simulink model "w31_v6"  (Simulink 7.9)
settings: Solver=FixedStepDiscrete  StartTime=0.0  StopTime=inf  FixedStep=0.01  RelTol=1e-3
undefined symbols (not defined in the file): DiscIntNeverNeededParam, magnitude
libraries: canmsglib x24, cansrvlib x22, simulink x12, iohwablib x5, legionoslib x3, ccpsrvlib x2, memsrvlib x1, tgttoollib x1, udssrvlib x1, wdgmlib x1
(part 3 of 5)

== system w31_v6/CAN_Receive_10ms/Remote_Control_CAN/remote_shake1 ==
  note: 内侧车轮转角30度，此处以内侧车轮为准，所以输出车轮转角为-30度到+30度
      | 车速范围为0-80km/h，纵向控制遥感往前推是加速
      | 制动压力范围0-8mpa，纵向控制遥感往后推是制动
  msg : Inport
  Function : TriggerPort  TriggerType=function-call  PortDimensions=1
  Accelerate : Subsystem  TreatAsAtomicUnit=on
  Constant : Constant  OutDataTypeStr=uint8  SampleTime=-1
  Decelerate : Subsystem  TreatAsAtomicUnit=on
  Gain : Gain  Gain=30/450
  If : If
  Memory : Memory  InheritSampleTime=on
  Merge : Merge
  Merge1 : Merge
  Remote_control_Io : canmsglib/CAN Unpack  CANdbFile=E:\matlab_ws\2012_Matlab_Vcu\w_serial\w3\w32\dbc\w32_CAN1_500kbs_0309_v5.dbc  MsgList=Remote_Control_Shake_2  MsgName=Remote_Control_Shake_2  MsgIDType=Standard (11-bit identifier)  MsgIdentifier=267  MsgLength=8  SignalInfo=Remote_X1_Reserved$48$16$1$1$1$0$1$0$-450$450$#Remote_X2_Lateral_Control$0$16$1$1$1$0$1$0$-450$450$#Remote_Y1_Longitudinal_Control$32$16$1$1$1$0$1$0$-450$450$#Remote_Y2_Reserved$16$16$1$1$1$0$-1$0$-450$450$#  NSignals=4  IDPort=off  TimestampPort=off  ErrorPort=off  RemotePort=off  LengthPort=off  StatusPort=off  StartBits=str2num('[int32(48);int32(0);int32(32);int32(16)]')  SignalSizes=str2num('[int32(16);int32(16);int32(16);int32(16)]')  ByteOrders=str2num('[int32(1);int32(1);int32(1);int32(1)]')  DataTypes=str2num('[int32(1);int32(1);int32(1);int32(1)]')  MultiplexTypes=str2num('[int32(1);int32(1);int32(1);int32(1)]')  MultiplexValues=str2num('[double(0);double(0);double(0);double(0)]')  Factors=str2num('[double(1);double(1);double(1);double(-1)]')  Offsets=str2num('[double(0);double(0);double(0);double(0)]')  Minimums=str2num('[double(-450);double(-450);double(-450);double(-450)]')  Maximums=str2num('[double(450);double(450);double(450);double(450)]')
      settings: DataFormat=CANdb specified signals
  Sum : Sum  Inputs=|++  OutDataTypeStr=uint8
  Terminator1 : Terminator
  Terminator3 : Terminator
  Remote_Power_Required : Outport
  Remote_Brake_Pressure_Required : Outport  Port=2
  Remote_Steering_Angle_Required : Outport  Port=3
  Remote_stutas : Outport  Port=4
  wires:
  Memory/1 -> Sum/2
  Sum/1 -> Memory/1, Remote_stutas/1
  Constant/1 -> Sum/1
  msg/1 -> Remote_control_Io/1
  Remote_control_Io/1 -> Terminator3/1
  Remote_control_Io/2 -> Gain/1
  Gain/1 -> Remote_Steering_Angle_Required/1
  Remote_control_Io/3 -> Accelerate/1(Speed_Required), Decelerate/1(BrakePressureRequired), If/1
  If/1 -> Accelerate/Action
  If/2 -> Decelerate/Action
  Accelerate/1(RemoteSpeedRequired) -> Merge/1
  Decelerate/1(RemoteSpeedRequired) -> Merge/2
  Accelerate/2(RemoteBrakePressureRequired) -> Merge1/1
  Decelerate/2(RemoteBrakePressureRequired) -> Merge1/2
  Merge/1 -> Remote_Power_Required/1
  Merge1/1 -> Remote_Brake_Pressure_Required/1
  Remote_control_Io/4 -> Terminator1/1

== system w31_v6/CAN_Receive_10ms/Remote_Control_CAN/shake_situation1 ==
  note: 输出1表示信号丢失
      | 输出0表示一切正常
  RxMsgCnt : Inport
  NoRxMsgCntMax : Inport  Port=2
  Chart : Stateflow chart  TreatAsAtomicUnit=on
  Relational Operator1 : RelationalOperator  Operator=~=  OutDataTypeStr=boolean
  Terminator : Terminator
  Unit Delay1 : UnitDelay  SampleTime=-1
  NoRxMsgComfirm : Outport
  wires:
  NoRxMsgCntMax/1 -> Chart/2(NoRxMsgCntMax)
  Unit Delay1/1 -> Relational Operator1/1
  RxMsgCnt/1 -> Relational Operator1/2, Unit Delay1/1
  Relational Operator1/1 -> Chart/1(RxMsg)
  Chart/1(NoRxMsgComfirm) -> NoRxMsgComfirm/1
  Chart/2(NoRxMsgCnt) -> Terminator/1

== system w31_v6/CAN_Receive_10ms/Status_Cal/Subsystem ==
  note: 等于0则说明存在严重故障
  Remote : Inport
  Chassis : Inport  Port=2
  iECU : Inport  Port=3
  Hardware : Inport  Port=4
  Bus Creator : BusCreator  Inputs=1
  Bus Creator1 : BusCreator
  Bus Creator2 : BusCreator  Inputs=7
  Bus Creator3 : BusCreator  Inputs=1
  Bus Creator4 : BusCreator  Inputs=2
  Bus Selector : BusSelector  OutputSignals=Remote_Analog.Remote_Analog_Status,Remote_IO.Remote_IO_Status
  Bus Selector1 : BusSelector  OutputSignals=EPSF_Receive.EPSF_Status_NoRxMsg,EPSR_Receive.EPSR_Status_NoRxMsg,DBSF_Receive.DBSF_Status_NoRxMsg,FL_Motor_Receive.FL_Motor_Status_NoRxMsg,FR_Motor_Receive.FR_Motor_Status_NoRxMsg,RL_Motor_Receive.RL_Motor_Status_NoRxMsg,RR_Motor_Receive.RR_Motor_Status_NoRxMsg
  Bus Selector2 : BusSelector  OutputSignals=iECU_Status
  Bus Selector3 : BusSelector  OutputSignals=Key_Ig_Cmd,Eme_Stop_Cmd
  Compare To Zero : simulink/Logic and Bit Operations/Compare To Zero  relop===  OutDataTypeStr=uint8
  Logical Operator : Logic  Operator=OR  AllPortsSameDT=off  OutDataTypeStr=boolean
  Logical Operator1 : Logic  Operator=OR  Inputs=11  AllPortsSameDT=off  OutDataTypeStr=boolean
  Vehicle_State : Outport
  Vehicle_Ready : Outport  Port=2
  wires:
  Remote/1 -> Bus Selector/1
  Bus Selector/1 -> Logical Operator/1  "<Remote_Analog_Status>"
  Bus Selector/2 -> Logical Operator/2  "<Remote_IO_Status>"
  Chassis/1 -> Bus Selector1/1
  Logical Operator/1 -> Bus Creator/1, Logical Operator1/1  "Remote_Status"
  Bus Selector1/1 -> Bus Creator2/1, Logical Operator1/2  "<EPSF_Status_NoRxMsg>"
  Bus Selector1/2 -> Bus Creator2/2, Logical Operator1/3  "<EPSR_Status_NoRxMsg>"
  Bus Selector1/3 -> Bus Creator2/3, Logical Operator1/4  "<DBSF_Status_NoRxMsg>"
  Bus Selector1/4 -> Bus Creator2/5, Logical Operator1/6  "<FL_Motor_Status_NoRxMsg>"
  Bus Selector1/5 -> Bus Creator2/6, Logical Operator1/7  "<FR_Motor_Status_NoRxMsg>"
  Bus Selector1/6 -> Bus Creator2/7, Logical Operator1/8  "<RL_Motor_Status_NoRxMsg>"
  Bus Selector1/7 -> Logical Operator1/9, Bus Creator2/4  "<RR_Motor_Status_NoRxMsg>"
  iECU/1 -> Bus Selector2/1
  Bus Selector2/1 -> Bus Creator3/1, Logical Operator1/10  "<iECU_Status>"
  Hardware/1 -> Bus Selector3/1
  Bus Selector3/1 -> Bus Creator4/1, Compare To Zero/1  "<Key_Ig_Cmd>"
  Bus Selector3/2 -> Bus Creator4/2, Logical Operator1/5  "<Eme_Stop_Cmd>"
  Bus Creator/1 -> Bus Creator1/1  "Remote_Status"
  Bus Creator2/1 -> Bus Creator1/2  "Chassis_Status"
  Bus Creator3/1 -> Bus Creator1/3  "iECU_Status"
  Bus Creator4/1 -> Bus Creator1/4  "Hardware_Status"
  Bus Creator1/1 -> Vehicle_State/1
  Compare To Zero/1 -> Logical Operator1/11
  Logical Operator1/1 -> Vehicle_Ready/1

== system w31_v6/CAN_Receive_10ms/Status_Cal/Subsystem1 ==
  Vehicle_Ready : Inport
  Chassis : Inport  Port=2
  Hardware : Inport  Port=3
  Abs{,1..3} (4 alike) : Abs
  Add1 : Sum  Inputs=++++
  Bus Creator : BusCreator  Inputs=6
  Bus Selector1 : BusSelector  OutputSignals=EPSF_Receive.F_Tire_Angle_Feedback,EPSR_Receive.R_Tire_Angle_Feedback,DBSF_Receive.DBSF_HP_Pressure_Feedback,FL_Motor_Receive.FL_RPM_Feedback,FR_Motor_Receive.FR_RPM_Feedback,RL_Motor_Receive.RL_RPM_Feedback,RR_Motor_Receive.RR_RPM_Feedback
  Bus Selector3 : BusSelector  OutputSignals=Key_Ig_Cmd
  Gain1 : Gain  Gain=1/4
  To_rpm : Gain  Gain=(3.14*0.69*60)/1000
  Vehicle_Status : Outport
  wires:
  Hardware/1 -> Bus Selector3/1
  Chassis/1 -> Bus Selector1/1
  Bus Selector1/1 -> Bus Creator/2  "<F_Tire_Angle_Feedback>"
  Bus Selector1/2 -> Bus Creator/3  "<R_Tire_Angle_Feedback>"
  Bus Selector1/4 -> Abs/1  "<FL_RPM_Feedback>"
  Bus Selector1/5 -> Abs1/1  "<FR_RPM_Feedback>"
  Bus Selector1/6 -> Abs2/1  "<RL_RPM_Feedback>"
  Bus Selector1/7 -> Abs3/1  "<RR_RPM_Feedback>"
  Abs/1 -> Add1/1
  Abs1/1 -> Add1/2
  Abs2/1 -> Add1/3
  Abs3/1 -> Add1/4
  Add1/1 -> Gain1/1
  Gain1/1 -> To_rpm/1
  To_rpm/1 -> Bus Creator/5  "Vehicle_Speed"
  Vehicle_Ready/1 -> Bus Creator/1  "Vehicle_Ready"
  Bus Selector3/1 -> Bus Creator/6  "<Key_Ig_Cmd>"
  Bus Creator/1 -> Vehicle_Status/1
  Bus Selector1/3 -> Bus Creator/4  "<DBSF_HP_Pressure_Feedback>"

== system w31_v6/CAN_Receive_10ms/iECU_CAN/iECU ==
  note: 内侧车轮转角30度，此处以内侧车轮为准，所以输出车轮转角为-30度到+30度
      | 车速范围为0-80km/h，纵向控制遥感往前推是加速
      | 制动压力范围0-8mpa，纵向控制遥感往后推是制动
  msg : Inport
  Function : TriggerPort  TriggerType=function-call  PortDimensions=1
  Constant : Constant  OutDataTypeStr=uint8  SampleTime=-1
  Data Type Conversion1 : DataTypeConversion  OutDataTypeStr=uint8
  Data Type Conversion2 : DataTypeConversion  OutDataTypeStr=uint8
  Data Type Conversion3 : DataTypeConversion  OutDataTypeStr=double
  Data Type Conversion4 : DataTypeConversion  OutDataTypeStr=double
  Memory : Memory  InheritSampleTime=on
  Sum : Sum  Inputs=|++  OutDataTypeStr=uint8
  Terminator : Terminator
  Terminator1 : Terminator
  Terminator2 : Terminator
  iECU_Input : canmsglib/CAN Unpack  CANdbFile=D:\W31_workspace\w31_CAN1_500kbs_0618_v5.1.dbc  MsgList=iECU  MsgName=iECU  MsgIDType=Standard (11-bit identifier)  MsgIdentifier=268  MsgLength=8  SignalInfo=iECU_BrakePressure_Cmd$28$8$1$2$1$0$1.000000e-01$0$0$8$#iECU_Control_Request_Flag$0$1$1$2$1$0$1$0$0$1$#iECU_E_Gear_Request$1$2$1$2$1$0$1$0$0$2$#iECU_FTire_Angle_Cmd$8$10$1$2$1$0$1.000000e-01$-30$-30$30$#iECU_RTire_Angle_Cmd$18$10$1$2$1$0$1.000000e-01$-30$-30$30$#iECU_Reseved1$3$2$1$2$1$0$1$0$0$2$#iECU_Reseved2$5$3$1$2$1$0$1$0$0$7$#iECU_Reseved3$46$18$1$2$1$0$1$0$0$500$#iECU_Speed_Cmd$36$10$1$2$1$0$1.000000e-01$0$0$80$#  NSignals=9  IDPort=off  TimestampPort=off  ErrorPort=off  RemotePort=off  LengthPort=off  StatusPort=off  StartBits=str2num('[int32(28);int32(0);int32(1);int32(8);int32(18);int32(3);int32(5);int32(46);int32(36)]')  SignalSizes=str2num('[int32(8);int32(1);int32(2);int32(10);int32(10);int32(2);int32(3);int32(18);int32(10)]')  ByteOrders=str2num('[int32(1);int32(1);int32(1);int32(1);int32(1);int32(1);int32(1);int32(1);int32(1)]')  DataTypes=str2num('[int32(2);int32(2);int32(2);int32(2);int32(2);int32(2);int32(2);int32(2);int32(2)]')  MultiplexTypes=str2num('[int32(1);int32(1);int32(1);int32(1);int32(1);int32(1);int32(1);int32(1);int32(1)]')  MultiplexValues=str2num('[double(0);double(0);double(0);double(0);double(0);double(0);double(0);double(0);double(0)]')  Factors=str2num('[double(1.000000e-01);double(1);double(1);double(1.000000e-01);double(1.000000e-01);double(1);double(1);double(1);double(1.000000e-01)]')  Offsets=str2num('[double(0);double(0);double(0);double(-30);double(-30);double(0);double(0);double(0);double(0)]')  Minimums=str2num('[double(0);double(0);double(0);double(-30);double(-30);double(0);double(0);double(0);double(0)]')  Maximums=str2num('[double(8);double(1);double(2);double(30);double(30);double(2);double(7);double(500);double(80)]')
      settings: DataFormat=CANdb specified signals
  iECU_Brake_Pressure_Required : Outport
  iECU_Control_Flag : Outport  Port=2
  iECU_Gear_Required : Outport  Port=3
  iECU_FTire_Angle_Required : Outport  Port=4
  iECU_RTire_Angle_Required : Outport  Port=5
  iECU_Speed_Required : Outport  Port=6
  iECU_Stutas : Outport  Port=7
  wires:
  Memory/1 -> Sum/2
  Sum/1 -> Memory/1, iECU_Stutas/1
  Constant/1 -> Sum/1
  msg/1 -> iECU_Input/1
  Data Type Conversion1/1 -> iECU_Control_Flag/1
  Data Type Conversion2/1 -> iECU_Gear_Required/1
  Data Type Conversion3/1 -> iECU_FTire_Angle_Required/1
  Data Type Conversion4/1 -> iECU_RTire_Angle_Required/1
  iECU_Input/1 -> iECU_Brake_Pressure_Required/1  "iECU_Brake_Pressure_Required"
  iECU_Input/2 -> Data Type Conversion1/1  "iECU_Control_Flag"
  iECU_Input/3 -> Data Type Conversion2/1  "iECU_Gear_Required"
  iECU_Input/4 -> Data Type Conversion3/1  "iECU_FTire_Angle_Required"
  iECU_Input/5 -> Data Type Conversion4/1  "iECU_RTire_Angle_Required"
  iECU_Input/6 -> Terminator/1
  iECU_Input/9 -> iECU_Speed_Required/1  "iECU_Speed_Required"
  iECU_Input/7 -> Terminator1/1
  iECU_Input/8 -> Terminator2/1

== system w31_v6/CAN_Receive_10ms/iECU_CAN/shake_situation1 ==
  note: 输出1表示信号丢失
      | 输出0表示一切正常
  RxMsgCnt : Inport
  NoRxMsgCntMax : Inport  Port=2
  Chart : Stateflow chart  TreatAsAtomicUnit=on
  Relational Operator1 : RelationalOperator  Operator=~=  OutDataTypeStr=boolean
  Terminator : Terminator
  Unit Delay1 : UnitDelay  SampleTime=-1
  NoRxMsgComfirm : Outport
  wires:
  NoRxMsgCntMax/1 -> Chart/2(NoRxMsgCntMax)
  Unit Delay1/1 -> Relational Operator1/1
  RxMsgCnt/1 -> Relational Operator1/2, Unit Delay1/1
  Relational Operator1/1 -> Chart/1(RxMsg)
  Chart/1(NoRxMsgComfirm) -> NoRxMsgComfirm/1
  Chart/2(NoRxMsgCnt) -> Terminator/1

== system w31_v6/Logic_And_Algorithm/Remote_mode_with_control_0/Brake_calculation ==
  0_4Mpa : Saturate  UpperLimit=4  LowerLimit=0
  Constant : Constant  SampleTime=-1
  Constant1 : Constant  Value=2  SampleTime=-1
  Constant2 : Constant  Value=0  SampleTime=-1
  Constant3 : Constant  Value=0  SampleTime=-1
  Delay : Delay  DelayLength=100
  Gain : Gain  Gain=2
  Multiport Switch : MultiPortSwitch  DataPortOrder=Specify indices  DataPortIndices={0,2,1}  zeroidx=off
  Sum : Sum  Inputs=|++
  Switch : Switch  Criteria=u2 > Threshold
  Break_Req : Outport
  Remote_EPB_Req : Outport  Port=2
  wires:
  [Remote_Brake_Pressure_Required_0] -> Sum/1
  Gain/1 -> Sum/2
  Sum/1 -> 0_4Mpa/1
  0_4Mpa/1 -> Break_Req/1  "Break_Req"
  [No_Remote_CAN_Msg_Or_Emg_Button_0] -> Gain/1
  [EPB_Control_Mode_0] -> Multiport Switch/1
  Constant/1 -> Multiport Switch/2
  Constant1/1 -> Multiport Switch/3
  Constant2/1 -> Multiport Switch/4
  Switch/1 -> Remote_EPB_Req/1
  [Key_Ig_Cmd_0] -> Delay/1
  Constant3/1 -> Switch/3
  Multiport Switch/1 -> Switch/1  "Remote_EPB_Req"
  Delay/1 -> Switch/2

== system w31_v6/Logic_And_Algorithm/Remote_mode_with_control_0/Power_calculation ==
  note: 输入是前进、倒退，输出是四个电机分别的旋转方向
  Constant : Constant  OutDataTypeStr=uint8
  Constant1 : Constant  Value=-1  OutDataTypeStr=int16
  Constant2 : Constant  Value=0  OutDataTypeStr=uint8
  Data Type Conversion : DataTypeConversion  OutDataTypeStr=uint8
  Display{,1..3} (4 alike) : Display
  Multiport Switch : MultiPortSwitch  DataPortOrder=Specify indices  DataPortIndices={0,2,1}  zeroidx=off  OutDataTypeStr=double
  PID_Controller : Subsystem
  Product{,1..3} (4 alike) : Product  RndMeth=Zero
  Speed distribution strategy : Subsystem
  Power_FL : Outport
  Power_FR : Outport  Port=2
  Power_RL : Outport  Port=3
  Power_RR : Outport  Port=4
  wires:
  [Remote_Gear1_0] -> Data Type Conversion/1
  Data Type Conversion/1 -> Multiport Switch/1, Display2/1
  Constant/1 -> Multiport Switch/2
  Constant1/1 -> Multiport Switch/3
  Constant2/1 -> Multiport Switch/4
  Multiport Switch/1 -> Product/1, Product1/1, Product2/1, Product3/1, Display1/1  "Rotation_to_Motor"
  PID_Controller/1(Power_to_FL) -> Product/2, Display/1  "Power_to_FR_Motor"
  PID_Controller/2(Power_to_FR) -> Product1/2  "Power_to_FL_Motor"
  PID_Controller/3(Power_to_RL) -> Product2/2  "Power_to_RR_Motor"
  PID_Controller/4(Power_to_RR) -> Product3/2  "Power_to_RL_Motor"
  Speed distribution strategy/1(Speed_to_FL_PID) -> PID_Controller/1(Desired_Speed_To_FL)
  Speed distribution strategy/2(Speed_to_FR_PID) -> PID_Controller/2(Desired_Speed_To_FR)
  Speed distribution strategy/3(Speed_to_RL_PID) -> PID_Controller/3(Desired_Speed_To_RL)
  Speed distribution strategy/4(Speed_to_RR_PID) -> PID_Controller/4(Desired_Speed_To_RR)
  Product/1 -> Power_FL/1  "Power_FL"
  Product1/1 -> Power_FR/1  "Power_FR"
  Product2/1 -> Power_RL/1  "Power_RL"
  Product3/1 -> Power_RR/1  "Power_RR"

== system w31_v6/Logic_And_Algorithm/Remote_mode_with_control_0/Signal_Input ==
  Chassis_CAN_input : Inport
  Sensor_CAN_input : Inport  Port=2
  Remote_CAN_input : Inport  Port=3
  Hardware_input : Inport  Port=4
  No_Remote_CAN_Msg_Or_Emg_Button : Inport  Port=5
  Chassis_Signal_Goto : Subsystem
  Emg_No_Msg : Subsystem
  Hardware_Signal_Goto1 : Subsystem
  Remote_Signal_Goto : Subsystem
  Terminator1 : Terminator
  wires:
  Chassis_CAN_input/1 -> Chassis_Signal_Goto/1(Chassis_Receive_input)
  Sensor_CAN_input/1 -> Terminator1/1
  Hardware_input/1 -> Hardware_Signal_Goto1/1(Hardware_input)
  Remote_CAN_input/1 -> Remote_Signal_Goto/1(Remote_CAN_input)
  No_Remote_CAN_Msg_Or_Emg_Button/1 -> Emg_No_Msg/1(No_Remote_CAN_Msg_Or_Emg_Button)

== system w31_v6/Logic_And_Algorithm/Remote_mode_with_control_0/Steering_calculation ==
  note: 前轮转角增大1.2倍
  Angle_Cal : Subsystem
  Angle_Control_Mode1 : Constant  Value=32  OutDataTypeStr=uint8
  F_Angle_Control_Mode : Constant  Value=32  OutDataTypeStr=uint8
  F_Angle_Rate : Constant  Value=500
  R_Angle_Rate : Constant  Value=500
  F_Steering_Angle : Outport
  R_Steering_Angle : Outport  Port=2
  F_Steering_Work_Mode : Outport  Port=3
  R_Steering_Work_Mode : Outport  Port=4
  F_Steering_Angle_Rate : Outport  Port=5
  R_Steering_Angle_Rate : Outport  Port=6
  wires:
  F_Angle_Control_Mode/1 -> F_Steering_Work_Mode/1  "F_Steering_Work_Mode"
  Angle_Cal/1(F_Steering_Angle) -> F_Steering_Angle/1  "F_Steering_Angle"
  Angle_Cal/2(R_Steering_Angle) -> R_Steering_Angle/1  "R_Steering_Angle"
  Angle_Control_Mode1/1 -> R_Steering_Work_Mode/1  "R_Steering_Work_Mode"
  F_Angle_Rate/1 -> F_Steering_Angle_Rate/1  "F_Steering_Angle_Rate"
  R_Angle_Rate/1 -> R_Steering_Angle_Rate/1  "R_Steering_Angle_Rate"

== system w31_v6/Logic_And_Algorithm/Remote_mode_with_control_2/Brake_calculation ==
  0_4Mpa : Saturate  UpperLimit=4  LowerLimit=0
  Compare To Constant : simulink/Logic and Bit Operations/Compare To Constant  relop=>=  const=650  OutDataTypeStr=uint8
  Constant : Constant  SampleTime=-1
  Constant1 : Constant  Value=2  SampleTime=-1
  Constant2 : Constant  Value=0  SampleTime=-1
  Constant3 : Constant  Value=0  SampleTime=-1
  Delay : Delay  DelayLength=100
  Gain : Gain  Gain=2
  Logical Operator : Logic  Operator=OR  AllPortsSameDT=off  OutDataTypeStr=boolean
  Multiport Switch : MultiPortSwitch  DataPortOrder=Specify indices  DataPortIndices={0,2,1}  zeroidx=off
  Sum : Sum  Inputs=|++
  Switch : Switch  Criteria=u2 > Threshold
  Break_Req : Outport
  Remote_EPB_Req : Outport  Port=2
  wires:
  Delay/1 -> Switch/2
  Multiport Switch/1 -> Switch/1  "Remote_EPB_Req"
  Constant3/1 -> Switch/3
  [Key_Ig_Cmd_2] -> Delay/1
  Switch/1 -> Remote_EPB_Req/1
  Constant2/1 -> Multiport Switch/4
  Constant1/1 -> Multiport Switch/3
  Constant/1 -> Multiport Switch/2
  [EPB_Control_Mode_2] -> Multiport Switch/1
  [No_Remote_CAN_Msg_Or_Emg_Button_2] -> Gain/1
  0_4Mpa/1 -> Break_Req/1  "Break_Req"
  Sum/1 -> 0_4Mpa/1
  Gain/1 -> Sum/2
  [Remote_Brake_Pressure_Required_2] -> Sum/1
  [Remote_Power_Required_2] -> Compare To Constant/1
  Compare To Constant/1 -> Logical Operator/1

== system w31_v6/Logic_And_Algorithm/Remote_mode_with_control_2/Power_calculation ==
  note: 输入是前进、倒退，输出是四个电机分别的旋转方向
  Constant : Constant  OutDataTypeStr=double
  Constant1 : Constant  Value=-1  OutDataTypeStr=double
  Constant2 : Constant  Value=0  OutDataTypeStr=double
  Data Type Conversion : DataTypeConversion  OutDataTypeStr=double
  Multiport Switch : MultiPortSwitch  DataPortOrder=Specify indices  DataPortIndices={0,2,1}  zeroidx=off  OutDataTypeStr=double
  PID_Controller : Subsystem
  Product{,1..3} (4 alike) : Product  RndMeth=Zero
  Speed distribution strategy : Subsystem
  Power_FL : Outport
  Power_FR : Outport  Port=2
  Power_RL : Outport  Port=3
  Power_RR : Outport  Port=4
  wires:
  Speed distribution strategy/3(Speed_to_RL_PID) -> PID_Controller/3(Desired_Speed_To_RL)
  Speed distribution strategy/4(Speed_to_RR_PID) -> PID_Controller/4(Desired_Speed_To_RR)
  Speed distribution strategy/1(Speed_to_FL_PID) -> PID_Controller/1(Desired_Speed_To_FL)
  Speed distribution strategy/2(Speed_to_FR_PID) -> PID_Controller/2(Desired_Speed_To_FR)
  [Remote_Gear1_2] -> Data Type Conversion/1
  Constant/1 -> Multiport Switch/2
  Constant1/1 -> Multiport Switch/3
  Constant2/1 -> Multiport Switch/4
  Multiport Switch/1 -> Product/1, Product2/1, Product3/1, Product1/1
  Data Type Conversion/1 -> Multiport Switch/1
  PID_Controller/1(Torque_to_FL_Motor) -> Product/2  "Power_to_FL_Motor"
  PID_Controller/2(Torque_to_FR_Motor) -> Product1/2  "Power_to_FR_Motor"
  Product1/1 -> Power_FR/1  "Power_FR"
  PID_Controller/3(Torque_to_RL_Motor) -> Product2/2  "Power_to_RL_Motor"
  Product2/1 -> Power_RL/1  "Power_RL"
  PID_Controller/4(Torque_to_RR_Motor) -> Product3/2  "Power_to_RR_Motor"
  Product3/1 -> Power_RR/1  "Power_RR"
  Product/1 -> Power_FL/1  "Power_FL"

== system w31_v6/Logic_And_Algorithm/Remote_mode_with_control_2/Signal_Input ==
  Remote_CAN_input : Inport
  Hardware_input : Inport  Port=2
  No_Remote_CAN_Msg_Or_Emg_Button : Inport  Port=3
  Emg_No_Msg : Subsystem
  Hardware_Signal_Goto1 : Subsystem
  Remote_Signal_Goto : Subsystem
  wires:
  No_Remote_CAN_Msg_Or_Emg_Button/1 -> Emg_No_Msg/1(No_Remote_CAN_Msg_Or_Emg_Button)
  Remote_CAN_input/1 -> Remote_Signal_Goto/1(Remote_CAN_input)
  Hardware_input/1 -> Hardware_Signal_Goto1/1(Hardware_input)

== system w31_v6/Logic_And_Algorithm/Remote_mode_with_control_2/Steering_calculation ==
  note: 前轮转角增大1.2倍
  Angle_Cal : Subsystem
  Angle_Control_Mode1 : Constant  Value=32  OutDataTypeStr=uint8
  F_Angle_Control_Mode : Constant  Value=32  OutDataTypeStr=uint8
  F_Angle_Rate : Constant  Value=500
  R_Angle_Rate : Constant  Value=500
  F_Steering_Angle : Outport
  R_Steering_Angle : Outport  Port=2
  F_Steering_Work_Mode : Outport  Port=3
  R_Steering_Work_Mode : Outport  Port=4
  F_Steering_Angle_Rate : Outport  Port=5
  R_Steering_Angle_Rate : Outport  Port=6
  wires:
  R_Angle_Rate/1 -> R_Steering_Angle_Rate/1  "R_Steering_Angle_Rate"
  F_Angle_Rate/1 -> F_Steering_Angle_Rate/1  "F_Steering_Angle_Rate"
  Angle_Control_Mode1/1 -> R_Steering_Work_Mode/1  "R_Steering_Work_Mode"
  Angle_Cal/2(R_Steering_Angle) -> R_Steering_Angle/1  "R_Steering_Angle"
  Angle_Cal/1(F_Steering_Angle) -> F_Steering_Angle/1  "F_Steering_Angle"
  F_Angle_Control_Mode/1 -> F_Steering_Work_Mode/1  "F_Steering_Work_Mode"

== system w31_v6/Logic_And_Algorithm/iECU_mode_with_control/Brake_calculation ==
  0_4Mpa : Saturate  UpperLimit=4  LowerLimit=0
  Gain : Gain  Gain=2
  Sum : Sum  Inputs=|+++
  Break_Req : Outport
  wires:
  [iECU_BrakePressureReq] -> Sum/1
  Sum/1 -> 0_4Mpa/1
  0_4Mpa/1 -> Break_Req/1  "Break_Req"
  [No_iECU_CAN_Msg_Or_Emg_Button] -> Gain/1
  Gain/1 -> Sum/3
  [iECU_RemoteBrakePressure] -> Sum/2

== system w31_v6/Logic_And_Algorithm/iECU_mode_with_control/Power_calculation ==
  note: 输入是前进、倒退，输出是四个电机分别的旋转方向
  Bus Creator1 : BusCreator
  Bus Creator2 : BusCreator
  PID_Controller : Subsystem
  PID_Reset_Cal : Subsystem
  Speed distribution strategy : Subsystem
  Subsystem : Subsystem
  Rotation_to_Motor_CANBus : Outport
  Torque_to_Motor_CANBus : Outport  Port=2
  wires:
  Bus Creator1/1 -> Rotation_to_Motor_CANBus/1  "Rotation_to_Motor_CANBus"
  Bus Creator2/1 -> Torque_to_Motor_CANBus/1  "Torque_to_Motor_CANBus"
  Speed distribution strategy/1(Speed_to_FR_PID) -> PID_Controller/1(Desired_Speed_To_FR)
  Speed distribution strategy/2(Speed_to_FL_PID) -> PID_Controller/2(Desired_Speed_To_FL1)
  Speed distribution strategy/3(Speed_to_RR_PID) -> PID_Controller/3(Desired_Speed_To_RR)
  Speed distribution strategy/4(Speed_to_RL_PID) -> PID_Controller/4(Desired_Speed_To_RL)
  Subsystem/1(Rotation_to_FL_Motor) -> Bus Creator1/1
  Subsystem/2(Rotation_to_FR_Motor) -> Bus Creator1/2
  Subsystem/3(Rotation_to_RL_Motor) -> Bus Creator1/3
  Subsystem/4(Rotation_to_RR_Motor) -> Bus Creator1/4
  PID_Controller/1(Torque_to_FR_Motor) -> Bus Creator2/1  "Torque_to_FR_Motor"
  PID_Controller/2(Torque_to_FL_Motor) -> Bus Creator2/2  "Torque_to_FL_Motor"
  PID_Controller/3(Torque_to_RR_Motor) -> Bus Creator2/3  "Torque_to_RR_Motor"
  PID_Controller/4(Torque_to_RL_Motor) -> Bus Creator2/4  "Torque_to_RL_Motor"

== system w31_v6/Logic_And_Algorithm/iECU_mode_with_control/Signal_Input ==
  Chassis_CAN_input : Inport
  Sensor_CAN_input : Inport  Port=2
  Remote_CAN_input : Inport  Port=3
  Hardware_input : Inport  Port=4
  iECU_CAN_input : Inport  Port=5
  No_iECU_CAN_Msg_Or_Emg_Button : Inport  Port=6
  Emg_No_Msg : Subsystem
  Hardware_Signal_Goto : Subsystem
  Remote_Signal_Goto : Subsystem
  Terminator : Terminator
  Terminator1 : Terminator
  iECU_Signal_Goto : Subsystem
  wires:
  Chassis_CAN_input/1 -> Hardware_Signal_Goto/1(Chassis_Receive_input)
  Sensor_CAN_input/1 -> Terminator1/1
  Hardware_input/1 -> Terminator/1
  Remote_CAN_input/1 -> Remote_Signal_Goto/1(Remote_CAN_input)
  iECU_CAN_input/1 -> iECU_Signal_Goto/1(iECU_CAN_input)
  No_iECU_CAN_Msg_Or_Emg_Button/1 -> Emg_No_Msg/1(No_iECU_CAN_Msg_Or_Emg_Button)

== system w31_v6/Logic_And_Algorithm/iECU_mode_with_control/Steering_calculation ==
  Angle_Control_Mode1 : Constant  Value=32  OutDataTypeStr=uint8
  F_Angle_Control_Mode : Constant  Value=32  OutDataTypeStr=uint8
  F_Angle_Rate : Constant  Value=500
  R_Angle_Rate : Constant  Value=500
  F_Steering_Angle : Outport
  R_Steering_Angle : Outport  Port=2
  F_Steering_Work_Mode : Outport  Port=3
  R_Steering_Work_Mode : Outport  Port=4
  F_Steering_Angle_Rate : Outport  Port=5
  R_Steering_Angle_Rate : Outport  Port=6
  wires:
  F_Angle_Control_Mode/1 -> F_Steering_Work_Mode/1  "F_Steering_Work_Mode"
  Angle_Control_Mode1/1 -> R_Steering_Work_Mode/1  "R_Steering_Work_Mode"
  F_Angle_Rate/1 -> F_Steering_Angle_Rate/1  "F_Steering_Angle_Rate"
  R_Angle_Rate/1 -> R_Steering_Angle_Rate/1  "R_Steering_Angle_Rate"
  [iECU_FTire_Angle_Rrquired] -> F_Steering_Angle/1
  [iECU_RTire_Angle_Rrquired] -> R_Steering_Angle/1

== system w31_v6/10ms_Signal_Output/SteerCAN_Out1/F/Subsystem ==
  deserved_angle : Inport
  Add1 : Sum
  Data Type Conversion : DataTypeConversion  OutDataTypeStr=uint8
  Data Type Conversion1 : DataTypeConversion  OutDataTypeStr=uint8
  Divide2 : Product  Inputs=*/
  Math Function2 : Math  Operator=mod  OutputSignalType=real  SaturateOnIntegerOverflow=on
  eps_angle_base : Constant  Value=256  OutDataTypeStr=double  SampleTime=-1
  eps_angle_init : Constant  Value=1024  OutDataTypeStr=Inherit: Inherit via back propagation  SampleTime=-1
  cmd_angle_high : Outport  OutDataTypeStr=uint8
  cmd_angle_low : Outport  Port=2  OutDataTypeStr=uint8
  wires:
  Add1/1 -> Math Function2/1, Divide2/1
  eps_angle_init/1 -> Add1/2
  eps_angle_base/1 -> Math Function2/2, Divide2/2
  Math Function2/1 -> Data Type Conversion1/1
  Divide2/1 -> Data Type Conversion/1
  Data Type Conversion/1 -> cmd_angle_high/1
  Data Type Conversion1/1 -> cmd_angle_low/1
  deserved_angle/1 -> Add1/1

== system w31_v6/10ms_Signal_Output/SteerCAN_Out1/R/Subsystem ==
  deserved_angle : Inport
  Add1 : Sum
  Data Type Conversion : DataTypeConversion  OutDataTypeStr=uint8
  Data Type Conversion1 : DataTypeConversion  OutDataTypeStr=uint8
  Divide2 : Product  Inputs=*/
  Math Function2 : Math  Operator=mod  OutputSignalType=real  SaturateOnIntegerOverflow=on
  eps_angle_base : Constant  Value=256  OutDataTypeStr=double  SampleTime=-1
  eps_angle_init : Constant  Value=1024  OutDataTypeStr=Inherit: Inherit via back propagation  SampleTime=-1
  cmd_angle_high : Outport  OutDataTypeStr=uint8
  cmd_angle_low : Outport  Port=2  OutDataTypeStr=uint8
  wires:
  Add1/1 -> Math Function2/1, Divide2/1
  eps_angle_init/1 -> Add1/2
  eps_angle_base/1 -> Math Function2/2, Divide2/2
  Math Function2/1 -> Data Type Conversion1/1
  Divide2/1 -> Data Type Conversion/1
  Data Type Conversion/1 -> cmd_angle_high/1
  Data Type Conversion1/1 -> cmd_angle_low/1
  deserved_angle/1 -> Add1/1

== system w31_v6/CAN_Receive_10ms/Hardware_Input/DI signal jittered/DI HS signal jitter1 ==
  DISig : Inport
  Compare To Zero : simulink/Logic and Bit Operations/Compare To Zero  relop=>  OutDataTypeStr=uint8
  Logical Operator : Logic  Inputs=3  AllPortsSameDT=off  OutDataTypeStr=boolean
  Logical Operator1 : Logic  Operator=OR  Inputs=3  AllPortsSameDT=off  OutDataTypeStr=boolean
  Memory{,1,5..6} (4 alike) : Memory  X0=1  InheritSampleTime=on
  Switch : Switch  Criteria=u2 ~= 0
  DISigJittered : Outport
  wires:
  Memory6/1 -> Logical Operator1/3
  Memory1/1 -> Logical Operator/3
  Switch/1 -> DISigJittered/1
  DISig/1 -> Compare To Zero/1
  Memory/1 -> Logical Operator/2, Memory1/1
  Memory5/1 -> Logical Operator1/2, Memory6/1
  Logical Operator/1 -> Switch/1
  Logical Operator1/1 -> Switch/3
  Compare To Zero/1 -> Logical Operator1/1, Memory5/1, Memory/1, Logical Operator/1, Switch/2

== system w31_v6/CAN_Receive_10ms/Hardware_Input/DI signal jittered/DI HS signal jitter2 ==
  DISig : Inport
  Compare To Zero : simulink/Logic and Bit Operations/Compare To Zero  relop=>  OutDataTypeStr=uint8
  Logical Operator : Logic  Inputs=3  AllPortsSameDT=off  OutDataTypeStr=boolean
  Logical Operator1 : Logic  Operator=OR  Inputs=3  AllPortsSameDT=off  OutDataTypeStr=boolean
  Memory{,1,5..6} (4 alike) : Memory  X0=1  InheritSampleTime=on
  Switch : Switch  Criteria=u2 ~= 0
  DISigJittered : Outport
  wires:
  Memory6/1 -> Logical Operator1/3
  Memory1/1 -> Logical Operator/3
  Switch/1 -> DISigJittered/1
  DISig/1 -> Compare To Zero/1
  Memory/1 -> Logical Operator/2, Memory1/1
  Memory5/1 -> Logical Operator1/2, Memory6/1
  Logical Operator/1 -> Switch/1
  Logical Operator1/1 -> Switch/3
  Compare To Zero/1 -> Logical Operator1/1, Memory5/1, Memory/1, Logical Operator/1, Switch/2

== system w31_v6/CAN_Receive_10ms/Hardware_Input/DI signal jittered/DI HS signal jitter3 ==
  DISig : Inport
  Compare To Zero : simulink/Logic and Bit Operations/Compare To Zero  relop=>  OutDataTypeStr=uint8
  Logical Operator : Logic  Inputs=3  AllPortsSameDT=off  OutDataTypeStr=boolean
  Logical Operator1 : Logic  Operator=OR  Inputs=3  AllPortsSameDT=off  OutDataTypeStr=boolean
  Memory{,1,5..6} (4 alike) : Memory  X0=1  InheritSampleTime=on
  Switch : Switch  Criteria=u2 ~= 0
  DISigJittered : Outport
  wires:
  Compare To Zero/1 -> Switch/2, Logical Operator/1, Memory/1, Memory5/1, Logical Operator1/1
  Logical Operator1/1 -> Switch/3
  Logical Operator/1 -> Switch/1
  Memory5/1 -> Memory6/1, Logical Operator1/2
  Memory/1 -> Memory1/1, Logical Operator/2
  DISig/1 -> Compare To Zero/1
  Switch/1 -> DISigJittered/1
  Memory1/1 -> Logical Operator/3
  Memory6/1 -> Logical Operator1/3

== system w31_v6/CAN_Receive_10ms/Hardware_Input/DI signal jittered/DI HS signal jitter8 ==
  DISig : Inport
  Compare To Zero : simulink/Logic and Bit Operations/Compare To Zero  relop=>  OutDataTypeStr=uint8
  Logical Operator : Logic  Inputs=3  AllPortsSameDT=off  OutDataTypeStr=boolean
  Logical Operator1 : Logic  Operator=OR  Inputs=3  AllPortsSameDT=off  OutDataTypeStr=boolean
  Memory{,1,5..6} (4 alike) : Memory  X0=1  InheritSampleTime=on
  Switch : Switch  Criteria=u2 ~= 0
  DISigJittered : Outport
  wires:
  Compare To Zero/1 -> Switch/2, Logical Operator/1, Memory/1, Memory5/1, Logical Operator1/1
  Logical Operator1/1 -> Switch/3
  Logical Operator/1 -> Switch/1
  Memory5/1 -> Memory6/1, Logical Operator1/2
  Memory/1 -> Memory1/1, Logical Operator/2
  DISig/1 -> Compare To Zero/1
  Switch/1 -> DISigJittered/1
  Memory1/1 -> Logical Operator/3
  Memory6/1 -> Logical Operator1/3

== system w31_v6/CAN_Receive_10ms/Remote_Control_CAN/remote_shake1/Accelerate ==
  note: 0-80kph
  Speed_Required : Inport
  Action Port : ActionPort  ActionType=then
  BrakePressureRequired : Constant  Value=0
  Gain : Gain  Gain=30/450
  To_rpm : Gain  Gain=1000/(3.14*0.53*60)
  RemoteSpeedRequired : Outport
  RemoteBrakePressureRequired : Outport  Port=2
  wires:
  BrakePressureRequired/1 -> RemoteBrakePressureRequired/1
  Speed_Required/1 -> Gain/1
  Gain/1 -> To_rpm/1
  To_rpm/1 -> RemoteSpeedRequired/1

== system w31_v6/CAN_Receive_10ms/Remote_Control_CAN/remote_shake1/Decelerate ==
  note: 0-4Mpa
  BrakePressureRequired : Inport
  Action Port : ActionPort  ActionType=else
  Gain : Gain  Gain=-4/450
  SpeedRequired : Constant  Value=0
  RemoteSpeedRequired : Outport
  RemoteBrakePressureRequired : Outport  Port=2
  wires:
  SpeedRequired/1 -> RemoteSpeedRequired/1
  BrakePressureRequired/1 -> Gain/1
  Gain/1 -> RemoteBrakePressureRequired/1

== system w31_v6/Logic_And_Algorithm/Remote_mode_with_control_0/Power_calculation/PID_Controller ==
  note: p调整为1.5
      | i调整为1
  Desired_Speed_To_FL : Inport
  Desired_Speed_To_FR : Inport  Port=2
  Desired_Speed_To_RL : Inport  Port=3
  Desired_Speed_To_RR : Inport  Port=4
  Power_to_FL : Outport
  Power_to_FR : Outport  Port=2
  Power_to_RL : Outport  Port=3
  Power_to_RR : Outport  Port=4
  wires:
  Desired_Speed_To_FL/1 -> Power_to_FL/1
  Desired_Speed_To_FR/1 -> Power_to_FR/1
  Desired_Speed_To_RL/1 -> Power_to_RL/1
  Desired_Speed_To_RR/1 -> Power_to_RR/1

== system w31_v6/Logic_And_Algorithm/Remote_mode_with_control_0/Power_calculation/Speed distribution strategy ==
  Data Type Conversion1 : DataTypeConversion
  Gain : Gain
  MATLAB Function : MATLAB Function  TreatAsAtomicUnit=on
  Switch{,1..3} (4 alike) : Switch  Criteria=u2 ~= 0
  Terminator : Terminator
  Terminator1 : Terminator
  motion distribution1 : Subsystem
  speed gear slection : MATLAB Function  TreatAsAtomicUnit=on
  Speed_to_FL_PID : Outport
  Speed_to_FR_PID : Outport  Port=2
  Speed_to_RL_PID : Outport  Port=3
  Speed_to_RR_PID : Outport  Port=4
  wires:
  [Remote_Gear2_0] -> Data Type Conversion1/1
  [Remote_Power_Required_0] -> speed gear slection/2(u2)
  Data Type Conversion1/1 -> speed gear slection/1(u1)
  motion distribution1/1(motion_f_dem) -> Terminator/1
  motion distribution1/2(motion_r_dem) -> Terminator1/1
  speed gear slection/1(y) -> motion distribution1/1(motion_dem), Gain/1
  [F_Steering_Angle] -> motion distribution1/2(steering angle_f_dem), MATLAB Function/1(delta_f)
  [R_Steering_Angle] -> motion distribution1/3(steering angle_r_dem), MATLAB Function/2(delta_r)
  [steering_mode_0] -> motion distribution1/4(drive mode), MATLAB Function/3(mode)
  motion distribution1/3(motion_fl_dem) -> Switch/3
  motion distribution1/4(motion_fr_dem) -> Switch1/3
  motion distribution1/5(motion_rl_dem) -> Switch2/3
  motion distribution1/6(motion_rr_dem) -> Switch3/3
  MATLAB Function/1(nan_code) -> Switch/2, Switch1/2, Switch2/2, Switch3/2
  Gain/1 -> Switch/1, Switch1/1, Switch2/1, Switch3/1
  Switch/1 -> Speed_to_FL_PID/1
  Switch1/1 -> Speed_to_FR_PID/1
  Switch2/1 -> Speed_to_RL_PID/1
  Switch3/1 -> Speed_to_RR_PID/1

== system w31_v6/Logic_And_Algorithm/Remote_mode_with_control_0/Signal_Input/Chassis_Signal_Goto ==
  Chassis_Receive_input : Inport
  Bus Selector3 : BusSelector  OutputSignals=FL_Motor_Receive.FL_RPM_Feedback,FR_Motor_Receive.FR_RPM_Feedback,RL_Motor_Receive.RL_RPM_Feedback,RR_Motor_Receive.RR_RPM_Feedback,DBSF_Receive.DBSF_Status_NoRxMsg,EPSF_Receive.F_Tire_Angle_Feedback,EPSR_Receive.R_Tire_Angle_Feedback
  tag scope: FL_RPM_Feedback=global, FR_RPM_Feedback=global, F_Steering_Angle=global, RL_RPM_Feedback=global, RR_RPM_Feedback=global, R_Steering_Angle=global
  wires:
  Bus Selector3/3 -> [RL_RPM_Feedback]  "<RL_RPM_Feedback>"
  Bus Selector3/2 -> [FR_RPM_Feedback]  "<FR_RPM_Feedback>"
  Bus Selector3/1 -> [FL_RPM_Feedback]  "<FL_RPM_Feedback>"
  Chassis_Receive_input/1 -> Bus Selector3/1
  Bus Selector3/4 -> [RR_RPM_Feedback]  "<RR_RPM_Feedback>"
  Bus Selector3/6 -> [F_Steering_Angle]  "<F_Tire_Angle_Feedback>"
  Bus Selector3/7 -> [R_Steering_Angle]  "<R_Tire_Angle_Feedback>"

== system w31_v6/Logic_And_Algorithm/Remote_mode_with_control_0/Signal_Input/Emg_No_Msg ==
  note: 15.5为轮端到EPS端的角传动比
  No_Remote_CAN_Msg_Or_Emg_Button : Inport
  Bus Selector3 : BusSelector  OutputSignals=No_Remote_CAN_Msg_Or_Emg_Button
  tag scope: No_Remote_CAN_Msg_Or_Emg_Button_0=global
  wires:
  Bus Selector3/1 -> [No_Remote_CAN_Msg_Or_Emg_Button_0]  "<No_Remote_CAN_Msg_Or_Emg_Button>"
  No_Remote_CAN_Msg_Or_Emg_Button/1 -> Bus Selector3/1

== system w31_v6/Logic_And_Algorithm/Remote_mode_with_control_0/Signal_Input/Hardware_Signal_Goto1 ==
  note: 15.5为轮端到EPS端的角传动比
  Hardware_input : Inport
  Bus Selector3 : BusSelector  OutputSignals=Eme_Stop_Cmd,Key_Ig_Cmd
  tag scope: Emg_Button_0=global, Key_Ig_Cmd_0=global
  wires:
  Bus Selector3/1 -> [Emg_Button_0]  "<Eme_Stop_Cmd>"
  Hardware_input/1 -> Bus Selector3/1
  Bus Selector3/2 -> [Key_Ig_Cmd_0]  "<Key_Ig_Cmd>"

== system w31_v6/Logic_And_Algorithm/Remote_mode_with_control_0/Signal_Input/Remote_Signal_Goto ==
  note: 15.5为轮端到EPS端的角传动比
  Remote_CAN_input : Inport
  Bus Selector3 : BusSelector  OutputSignals=Remote_Analog.Remote_Power_Required,Remote_Analog.Remote_Brake_Pressure_Required,Remote_Analog.Remote_Steering_Angle_Required,Remote_IO.Remote_Coordinate_System_Switch,Remote_IO.Remote_Steering_Mode_Switch1,Remote_IO.Remote_Gear1,Remote_IO.Remote_Gear2,Remote_IO.EPB_Control_Mode,Remote_IO.Remote_Steering_Mode_Switch2,Remote_IO.Remote_IO_Status,Remote_Analog.Remote_Analog_Status
  Logical Operator : Logic  Operator=OR  AllPortsSameDT=off  OutDataTypeStr=boolean
  Tire2EPS : Gain  Gain=15.5
  tag scope: EPB_Control_Mode_0=global, Remote_Brake_Pressure_Required_0=global, Remote_Coordinate_System_Switch_0=global, Remote_Gear1_0=global, Remote_Gear2_0=global, Remote_Power_Required_0=global, Remote_Status_0=global, Remote_Steering_Angle_Required_0=global, Remote_Steering_Mode_Switch1_0=global, Remote_Steering_Mode_Switch2_0=global
  wires:
  Logical Operator/1 -> [Remote_Status_0]
  Bus Selector3/11 -> Logical Operator/2  "<Remote_Analog_Status>"
  Bus Selector3/10 -> Logical Operator/1  "<Remote_IO_Status>"
  Tire2EPS/1 -> [Remote_Steering_Angle_Required_0]
  Bus Selector3/9 -> [Remote_Steering_Mode_Switch2_0]  "<Remote_Steering_Mode_Switch2>"
  Bus Selector3/8 -> [EPB_Control_Mode_0]  "<EPB_Control_Mode>"
  Bus Selector3/7 -> [Remote_Gear2_0]  "<Remote_Gear2>"
  Bus Selector3/6 -> [Remote_Gear1_0]  "<Remote_Gear1>"
  Bus Selector3/5 -> [Remote_Steering_Mode_Switch1_0]  "<Remote_Steering_Mode_Switch1>"
  Bus Selector3/4 -> [Remote_Coordinate_System_Switch_0]  "<Remote_Coordinate_System_Switch>"
  Remote_CAN_input/1 -> Bus Selector3/1
  Bus Selector3/1 -> [Remote_Power_Required_0]  "<Remote_Power_Required>"
  Bus Selector3/2 -> [Remote_Brake_Pressure_Required_0]  "<Remote_Brake_Pressure_Required>"
  Bus Selector3/3 -> Tire2EPS/1  "<Remote_Steering_Angle_Required>"

== system w31_v6/Logic_And_Algorithm/Remote_mode_with_control_0/Steering_calculation/Angle_Cal ==
  note: 前轮转角增大1.2倍
  Display : Display
  Drive_Mode_Switch_Case : SwitchCase  CaseConditions={0,3,2,4}
  F_Steer_mode : Subsystem  TreatAsAtomicUnit=on
  Merge : Merge  Inputs=5
  Merge1 : Merge  Inputs=5
  Parallel_Steer_mode : Subsystem
  R_Steer_mode : Subsystem
  Reverse_Steer_mode : Subsystem
  Steer_Model_Judge : Subsystem
  turn_in_place : Subsystem  TreatAsAtomicUnit=on
  F_Steering_Angle : Outport
  R_Steering_Angle : Outport  Port=2
  wires:
  Drive_Mode_Switch_Case/5 -> F_Steer_mode/Action
  Drive_Mode_Switch_Case/1 -> Parallel_Steer_mode/Action
  Drive_Mode_Switch_Case/2 -> Reverse_Steer_mode/Action
  Drive_Mode_Switch_Case/3 -> R_Steer_mode/Action
  Steer_Model_Judge/1(Steering_mode) -> Drive_Mode_Switch_Case/1
  Merge/1 -> F_Steering_Angle/1
  Merge1/1 -> R_Steering_Angle/1
  Parallel_Steer_mode/1(F_Steering_Angle) -> Merge/1
  Reverse_Steer_mode/1(F_Steering_Angle) -> Merge/2
  R_Steer_mode/1(F_Steering_Angle) -> Merge/3
  F_Steer_mode/1(F_Steering_Angle) -> Merge/4
  Parallel_Steer_mode/2(R_Steering_Angle) -> Merge1/1
  [Remote_Steering_Angle_Required_0] -> Parallel_Steer_mode/1(Remote_steering), Reverse_Steer_mode/1(Remote_steering), R_Steer_mode/1(Remote_steering), F_Steer_mode/1(Remote_steering), turn_in_place/1(Remote_steering), Display/1
  R_Steer_mode/2(R_Steering_Angle) -> Merge1/3
  F_Steer_mode/2(R_Steering_Angle) -> Merge1/4
  Reverse_Steer_mode/2(R_Steering_Angle) -> Merge1/2
  Drive_Mode_Switch_Case/4 -> turn_in_place/Action
  turn_in_place/1(F_Steering_Angle) -> Merge/5
  turn_in_place/2(R_Steering_Angle) -> Merge1/5

== system w31_v6/Logic_And_Algorithm/Remote_mode_with_control_2/Power_calculation/PID_Controller ==
  note: p调整为1.5
      | i调整为1
  Desired_Speed_To_FL : Inport
  Desired_Speed_To_FR : Inport  Port=2
  Desired_Speed_To_RL : Inport  Port=3
  Desired_Speed_To_RR : Inport  Port=4
  Torque_to_FL_Motor : Outport
  Torque_to_FR_Motor : Outport  Port=2
  Torque_to_RL_Motor : Outport  Port=3
  Torque_to_RR_Motor : Outport  Port=4
  wires:
  Desired_Speed_To_FR/1 -> Torque_to_FR_Motor/1
  Desired_Speed_To_FL/1 -> Torque_to_FL_Motor/1
  Desired_Speed_To_RR/1 -> Torque_to_RR_Motor/1
  Desired_Speed_To_RL/1 -> Torque_to_RL_Motor/1

== system w31_v6/Logic_And_Algorithm/Remote_mode_with_control_2/Power_calculation/Speed distribution strategy ==
  note: 注意！！！此处的输出顺序和电机顺序不一致
  Data Type Conversion1 : DataTypeConversion
  Gain : Gain  Gain=0.3
  Product{1..4} (4 alike) : Product  RndMeth=Zero
  Saturation : Saturate  UpperLimit=1  LowerLimit=-1
  speed gear slection : MATLAB Function  TreatAsAtomicUnit=on
  truin_in_place_gain : MATLAB Function  TreatAsAtomicUnit=on
  Speed_to_FL_PID : Outport
  Speed_to_FR_PID : Outport  Port=2
  Speed_to_RL_PID : Outport  Port=3
  Speed_to_RR_PID : Outport  Port=4
  wires:
  [Remote_Power_Required_2] -> Gain/1
  [Remote_Steering_Angle_Required_2] -> Saturation/1
  [steering_drive_mode2] -> truin_in_place_gain/1(mode)
  Saturation/1 -> truin_in_place_gain/2(steer_angle)
  Product2/1 -> Speed_to_FR_PID/1
  Product1/1 -> Speed_to_FL_PID/1
  Product4/1 -> Speed_to_RR_PID/1
  Product3/1 -> Speed_to_RL_PID/1
  truin_in_place_gain/1(gain1) -> Product1/1
  truin_in_place_gain/2(gain2) -> Product2/1
  truin_in_place_gain/3(gain3) -> Product3/1
  truin_in_place_gain/4(gain4) -> Product4/1
  [Remote_Gear2_2] -> Data Type Conversion1/1
  Data Type Conversion1/1 -> speed gear slection/1(u1)
  Gain/1 -> speed gear slection/2(u2)
  speed gear slection/1(y) -> Product4/2, Product3/2, Product2/2, Product1/2

== system w31_v6/Logic_And_Algorithm/Remote_mode_with_control_2/Signal_Input/Emg_No_Msg ==
  note: 15.5为轮端到EPS端的角传动比
  No_Remote_CAN_Msg_Or_Emg_Button : Inport
  Bus Selector3 : BusSelector  OutputSignals=No_Remote_CAN_Msg_Or_Emg_Button
  tag scope: No_Remote_CAN_Msg_Or_Emg_Button_2=global
  wires:
  No_Remote_CAN_Msg_Or_Emg_Button/1 -> Bus Selector3/1
  Bus Selector3/1 -> [No_Remote_CAN_Msg_Or_Emg_Button_2]  "<No_Remote_CAN_Msg_Or_Emg_Button>"

== system w31_v6/Logic_And_Algorithm/Remote_mode_with_control_2/Signal_Input/Hardware_Signal_Goto1 ==
  note: 15.5为轮端到EPS端的角传动比
  Hardware_input : Inport
  Bus Selector3 : BusSelector  OutputSignals=Eme_Stop_Cmd,Key_Ig_Cmd
  tag scope: Emg_Button_2=global, Key_Ig_Cmd_2=global
  wires:
  Bus Selector3/2 -> [Key_Ig_Cmd_2]  "<Key_Ig_Cmd>"
  Hardware_input/1 -> Bus Selector3/1
  Bus Selector3/1 -> [Emg_Button_2]  "<Eme_Stop_Cmd>"

== system w31_v6/Logic_And_Algorithm/Remote_mode_with_control_2/Signal_Input/Remote_Signal_Goto ==
  note: 15.5为轮端到EPS端的角传动比
  Remote_CAN_input : Inport
  Bus Selector3 : BusSelector  OutputSignals=Remote_Analog.Remote_Power_Required,Remote_Analog.Remote_Brake_Pressure_Required,Remote_Analog.Remote_Steering_Angle_Required,Remote_IO.Remote_Coordinate_System_Switch,Remote_IO.Remote_Steering_Mode_Switch1,Remote_IO.Remote_Gear1,Remote_IO.Remote_Gear2,Remote_IO.EPB_Control_Mode,Remote_IO.Remote_Steering_Mode_Switch2,Remote_IO.Remote_IO_Status,Remote_Analog.Remote_Analog_Status
  Logical Operator : Logic  Operator=OR  AllPortsSameDT=off  OutDataTypeStr=boolean
  Tire2EPS : Gain  Gain=15.5
  tag scope: EPB_Control_Mode_2=global, Remote_Brake_Pressure_Required_2=global, Remote_Coordinate_System_Switch_2=global, Remote_Gear1_2=global, Remote_Gear2_2=global, Remote_Power_Required_2=global, Remote_Status_2=global, Remote_Steering_Angle_Required_2=global, Remote_Steering_Mode_Switch1_2=global, Remote_Steering_Mode_Switch2_2=global
  wires:
  Logical Operator/1 -> [Remote_Status_2]
  Bus Selector3/11 -> Logical Operator/2  "<Remote_Analog_Status>"
  Bus Selector3/10 -> Logical Operator/1  "<Remote_IO_Status>"
  Tire2EPS/1 -> [Remote_Steering_Angle_Required_2]
  Bus Selector3/9 -> [Remote_Steering_Mode_Switch2_2]  "<Remote_Steering_Mode_Switch2>"
  Bus Selector3/8 -> [EPB_Control_Mode_2]  "<EPB_Control_Mode>"
  Bus Selector3/7 -> [Remote_Gear2_2]  "<Remote_Gear2>"
  Bus Selector3/6 -> [Remote_Gear1_2]  "<Remote_Gear1>"
  Bus Selector3/5 -> [Remote_Steering_Mode_Switch1_2]  "<Remote_Steering_Mode_Switch1>"
  Bus Selector3/4 -> [Remote_Coordinate_System_Switch_2]  "<Remote_Coordinate_System_Switch>"
  Remote_CAN_input/1 -> Bus Selector3/1
  Bus Selector3/1 -> [Remote_Power_Required_2]  "<Remote_Power_Required>"
  Bus Selector3/2 -> [Remote_Brake_Pressure_Required_2]  "<Remote_Brake_Pressure_Required>"
  Bus Selector3/3 -> Tire2EPS/1  "<Remote_Steering_Angle_Required>"

== system w31_v6/Logic_And_Algorithm/Remote_mode_with_control_2/Steering_calculation/Angle_Cal ==
  note: 前轮转角增大1.2倍
  Drive_Mode_Switch_Case : SwitchCase  CaseConditions={0,3,2,4}
  F_Steer_mode : Subsystem  TreatAsAtomicUnit=on
  Merge : Merge  Inputs=5
  Merge1 : Merge  Inputs=5
  Parallel_Steer_mode : Subsystem
  R_Steer_mode : Subsystem
  Reverse_Steer_mode : Subsystem
  Steer_Model_Judge : Subsystem
  turn_in_place : Subsystem  TreatAsAtomicUnit=on
  F_Steering_Angle : Outport
  R_Steering_Angle : Outport  Port=2
  wires:
  Reverse_Steer_mode/2(R_Steering_Angle) -> Merge1/2
  F_Steer_mode/2(R_Steering_Angle) -> Merge1/4
  R_Steer_mode/2(R_Steering_Angle) -> Merge1/3
  [Remote_Steering_Angle_Required_2] -> Parallel_Steer_mode/1(Remote_steering), Reverse_Steer_mode/1(Remote_steering), R_Steer_mode/1(Remote_steering), F_Steer_mode/1(Remote_steering), turn_in_place/1(Remote_steering)
  Parallel_Steer_mode/2(R_Steering_Angle) -> Merge1/1
  F_Steer_mode/1(F_Steering_Angle) -> Merge/4
  R_Steer_mode/1(F_Steering_Angle) -> Merge/3
  Reverse_Steer_mode/1(F_Steering_Angle) -> Merge/2
  Parallel_Steer_mode/1(F_Steering_Angle) -> Merge/1
  Merge1/1 -> R_Steering_Angle/1
  Merge/1 -> F_Steering_Angle/1
  Steer_Model_Judge/1(Steering_model) -> Drive_Mode_Switch_Case/1
  Drive_Mode_Switch_Case/3 -> R_Steer_mode/Action
  Drive_Mode_Switch_Case/2 -> Reverse_Steer_mode/Action
  Drive_Mode_Switch_Case/1 -> Parallel_Steer_mode/Action
  Drive_Mode_Switch_Case/5 -> F_Steer_mode/Action
  Drive_Mode_Switch_Case/4 -> turn_in_place/Action
  turn_in_place/1(F_Steering_Angle) -> Merge/5
  turn_in_place/2(R_Steering_Angle) -> Merge1/5

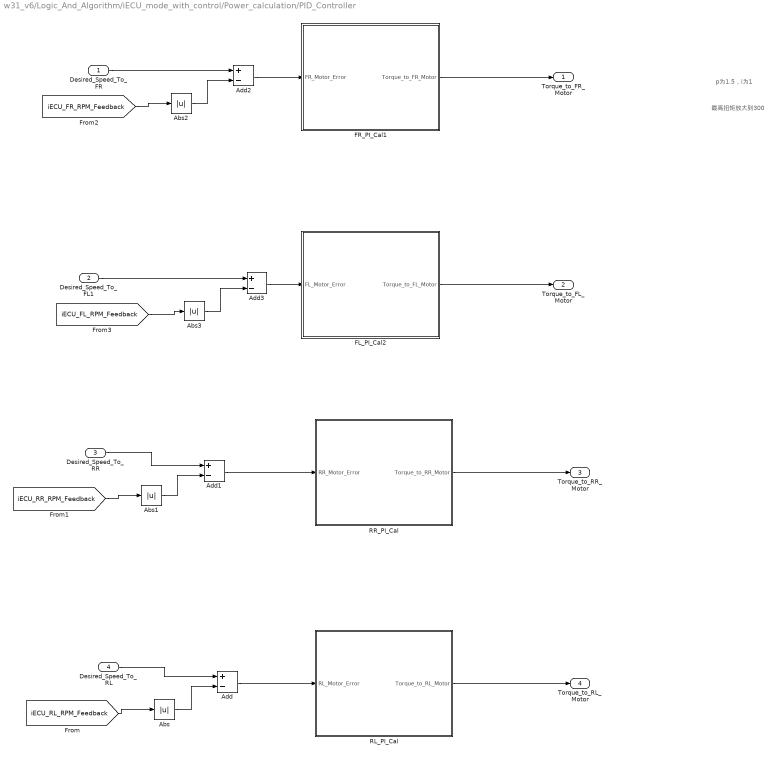
== system w31_v6/Logic_And_Algorithm/iECU_mode_with_control/Power_calculation/PID_Controller ==
  note: p为1.5，i为1
  note: 最高扭矩放大到300
  Desired_Speed_To_FR : Inport
  Desired_Speed_To_FL1 : Inport  Port=2
  Desired_Speed_To_RR : Inport  Port=3
  Desired_Speed_To_RL : Inport  Port=4
  Abs{,1..3} (4 alike) : Abs
  Add{,1..3} (4 alike) : Sum  Inputs=+-
  FL_PI_Cal2 : Subsystem
  FR_PI_Cal1 : Subsystem
  RL_PI_Cal : Subsystem
  RR_PI_Cal : Subsystem
  Torque_to_FR_Motor : Outport
  Torque_to_FL_Motor : Outport  Port=2
  Torque_to_RR_Motor : Outport  Port=3
  Torque_to_RL_Motor : Outport  Port=4
  wires:
  FR_PI_Cal1/1(Torque_to_FR_Motor) -> Torque_to_FR_Motor/1
  RL_PI_Cal/1(Torque_to_RL_Motor) -> Torque_to_RL_Motor/1
  RR_PI_Cal/1(Torque_to_RR_Motor) -> Torque_to_RR_Motor/1
  FL_PI_Cal2/1(Torque_to_FL_Motor) -> Torque_to_FL_Motor/1
  [iECU_RL_RPM_Feedback] -> Abs/1
  Desired_Speed_To_RL/1 -> Add/1
  Abs/1 -> Add/2
  Add/1 -> RL_PI_Cal/1(RL_Motor_Error)
  [iECU_RR_RPM_Feedback] -> Abs1/1
  Abs1/1 -> Add1/2
  Desired_Speed_To_RR/1 -> Add1/1
  Add1/1 -> RR_PI_Cal/1(RR_Motor_Error)
  [iECU_FR_RPM_Feedback] -> Abs2/1
  Abs2/1 -> Add2/2
  Desired_Speed_To_FR/1 -> Add2/1
  Add2/1 -> FR_PI_Cal1/1(FR_Motor_Error)
  [iECU_FL_RPM_Feedback] -> Abs3/1
  Abs3/1 -> Add3/2
  Desired_Speed_To_FL1/1 -> Add3/1
  Add3/1 -> FL_PI_Cal2/1(FL_Motor_Error)

== system w31_v6/Logic_And_Algorithm/iECU_mode_with_control/Power_calculation/PID_Reset_Cal ==
  Add : Sum
  Compare To Constant : simulink/Logic and Bit Operations/Compare To Constant  relop===  const=2  OutDataTypeStr=uint8
  Compare To Constant1 : simulink/Logic and Bit Operations/Compare To Constant  relop=>=  const=8  OutDataTypeStr=uint8
  Compare To Constant2 : simulink/Logic and Bit Operations/Compare To Constant  relop=<=  const=0.5  OutDataTypeStr=uint8
  Logical Operator : Logic  Operator=OR  Inputs=4  AllPortsSameDT=off  OutDataTypeStr=boolean
  tag scope: iECU_PID_Reset=global
  wires:
  [iECU_GearRequestAfterCal] -> Compare To Constant/1
  [No_iECU_CAN_Msg_Or_Emg_Button] -> Logical Operator/2
  Compare To Constant/1 -> Logical Operator/1
  Logical Operator/1 -> [iECU_PID_Reset]
  [iECU_BrakePressureReq] -> Add/1
  [iECU_RemoteBrakePressure] -> Add/2
  Add/1 -> Compare To Constant1/1
  Compare To Constant1/1 -> Logical Operator/3
  [iECU_SpeedReq] -> Compare To Constant2/1
  Compare To Constant2/1 -> Logical Operator/4

== system w31_v6/Logic_And_Algorithm/iECU_mode_with_control/Power_calculation/Speed distribution strategy ==
  Data Type Conversion : DataTypeConversion
  MATLAB Function : MATLAB Function  TreatAsAtomicUnit=on
  kph2rpm : Gain  Gain=1000/(3.14*0.53*60)
  Speed_to_FR_PID : Outport
  Speed_to_FL_PID : Outport  Port=2
  Speed_to_RR_PID : Outport  Port=3
  Speed_to_RL_PID : Outport  Port=4
  wires:
  [iECU_SpeedLimReq] -> Data Type Conversion/1
  [iECU_SpeedReq] -> MATLAB Function/2(u2)
  Data Type Conversion/1 -> MATLAB Function/1(u1)
  MATLAB Function/1(y) -> kph2rpm/1
  kph2rpm/1 -> Speed_to_FR_PID/1, Speed_to_FL_PID/1, Speed_to_RR_PID/1, Speed_to_RL_PID/1
